simulink model "case_study_2"  (R2022a)
settings: Solver=VariableStepAuto  StartTime=0.0  StopTime=2000  RelTol=1e-3
settings Model: Creator=spinolam  LastModifiedBy=spinolam

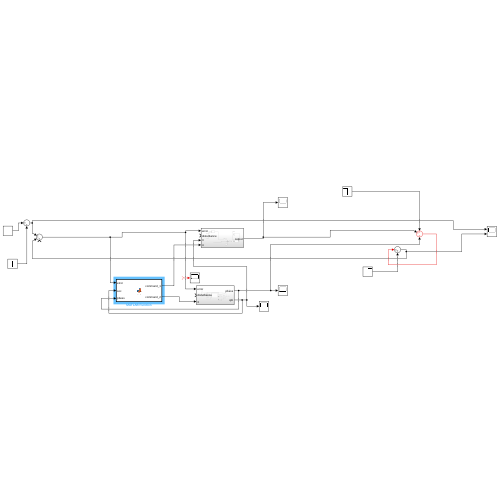
[thumbnail: Simulink's stored preview of the top-level diagram]
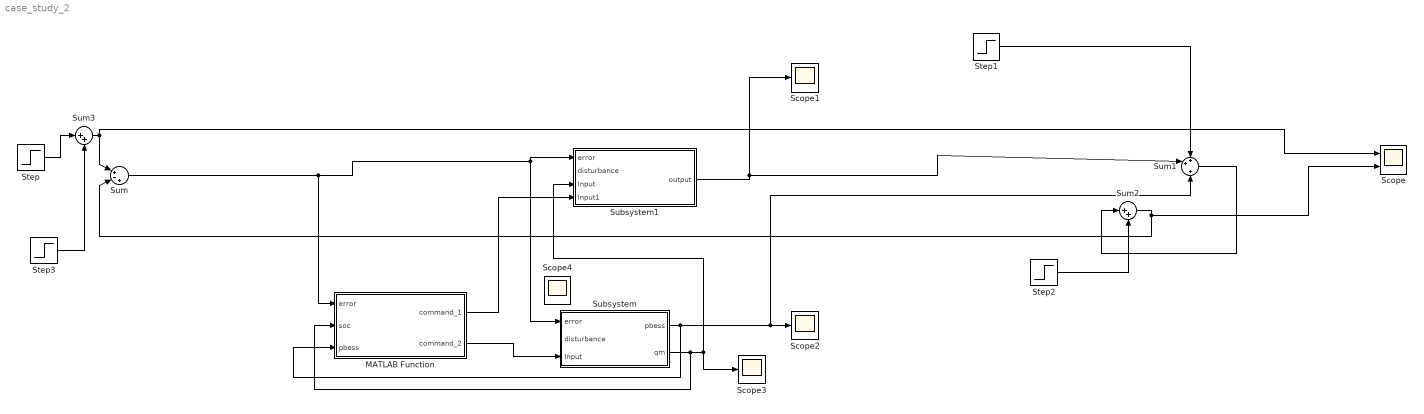
== system case_study_2 ==
  MATLAB Function : MATLAB Function  TreatAsAtomicUnit=on
  Scope : Scope  NumInputPorts=2
  Scope{1..4} (4 alike) : Scope
  Step : Step  Time=20  Before=1000  After=1300
  Step1 : Step  Time=100  After=-200
  Step2 : Step  Time=200  After=100
  Step3 : Step  Time=400  After=-100
  Subsystem : Subsystem
  Subsystem1 : Subsystem
  Sum : Sum  Inputs=|+-+
  Sum1 : Sum  Inputs=++|+
  Sum2 : Sum  Inputs=|++
  Sum3 : Sum  Inputs=|++
  wires:
  Step1/1 -> Sum1/1
  Sum1/1 -> Sum2/1
  Sum/1 -> MATLAB Function/1(error), Subsystem/1(error), Subsystem1/1(error)
  Subsystem1/1(output) -> Scope1/1, Sum1/2
  Subsystem/1(pbess) -> MATLAB Function/3(pbess), Sum1/3, Scope2/1
  Subsystem/2(qm) -> MATLAB Function/2(soc), Scope3/1, Subsystem1/3(Input)
  Sum2/1 -> Scope/2, Sum/2
  Step2/1 -> Sum2/2
  ? -> Scope4/1
  MATLAB Function/2(command_2) -> Subsystem/3(Input)
  MATLAB Function/1(command_1) -> Subsystem1/4(Input1)
  Step/1 -> Sum3/1
  Step3/1 -> Sum3/2
  Sum3/1 -> Sum/1, Scope/1

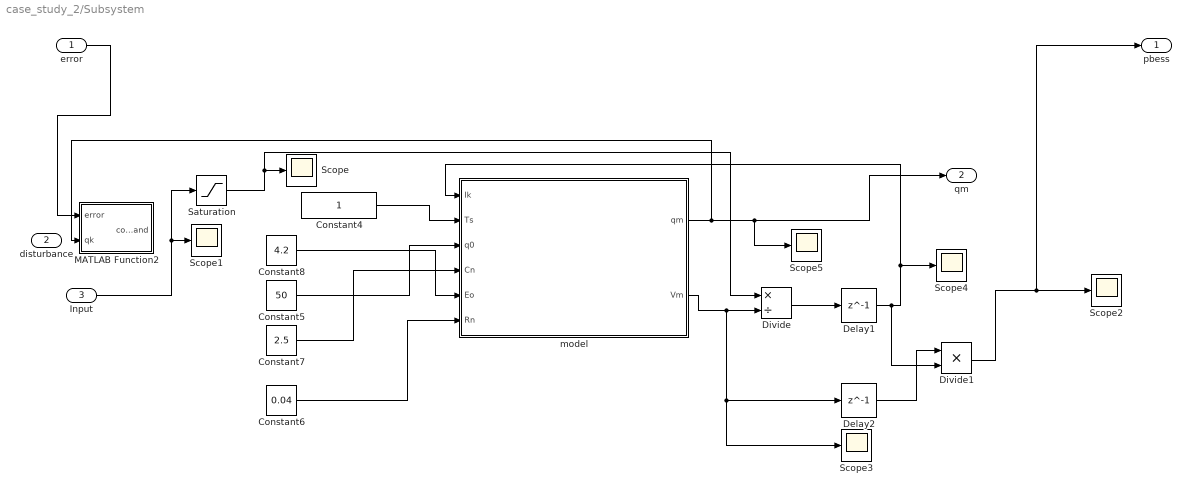
== system case_study_2/Subsystem ==
  error : Inport
  disturbance : Inport  Port=2
  Input : Inport  Port=3
  Constant4 : Constant  SampleTime=1
  Constant5 : Constant  Value=50
  Constant6 : Constant  Value=0.04
  Constant7 : Constant  Value=2.5
  Constant8 : Constant  Value=4.2
  Delay1 : Delay  DelayLength=1  InitialCondition=0  SampleTime=1
  Delay2 : Delay  DelayLength=1  InitialCondition=0  SampleTime=1
  Divide : Product  Inputs=*/
  Divide1 : Product  Inputs=**
  MATLAB Function2 : MATLAB Function  TreatAsAtomicUnit=on
  Saturation : Saturate  UpperLimit=140  LowerLimit=-140
  Scope{,1..5} (6 alike) : Scope
  model : MATLAB Function  TreatAsAtomicUnit=on  SystemSampleTime=1
  pbess : Outport
  qm : Outport  Port=2
  wires:
  Constant4/1 -> model/2(Ts)
  Constant6/1 -> model/6(Rn)
  Delay1/1 -> Divide1/2, Scope4/1, model/1(Ik)
  Divide1/1 -> pbess/1, Scope2/1
  Constant7/1 -> model/4(Cn)
  Divide/1 -> Delay1/1
  Delay2/1 -> Divide1/1
  Constant8/1 -> model/5(Eo)
  error/1 -> MATLAB Function2/1(error)
  model/2(Vm) -> Scope3/1, Delay2/1, Divide/2
  Constant5/1 -> model/3(q0)
  model/1(qm) -> MATLAB Function2/2(qk), Scope5/1, qm/1
  Saturation/1 -> Scope/1, Divide/1
  Input/1 -> Scope1/1, Saturation/1

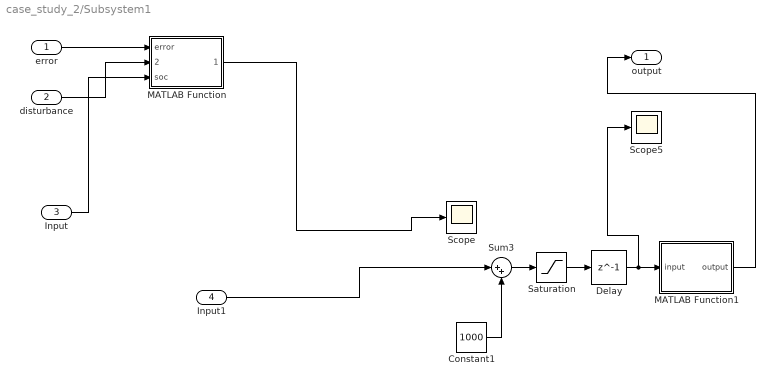
== system case_study_2/Subsystem1 ==
  error : Inport
  disturbance : Inport  Port=2
  Input : Inport  Port=3
  Input1 : Inport  Port=4
  Constant1 : Constant  Value=1000
  Delay : Delay  DelayLength=1  InitialCondition=1000  SampleTime=1
  MATLAB Function : MATLAB Function  TreatAsAtomicUnit=on
  MATLAB Function1 : MATLAB Function  TreatAsAtomicUnit=on
  Saturation : Saturate  UpperLimit=1500  LowerLimit=1000
  Scope : Scope
  Scope5 : Scope
  Sum3 : Sum  Inputs=|++
  output : Outport
  wires:
  MATLAB Function1/1(output) -> output/1
  MATLAB Function/1(command) -> Scope/1
  error/1 -> MATLAB Function/1(error)
  disturbance/1 -> MATLAB Function/2(disturbance)
  Sum3/1 -> Saturation/1
  Delay/1 -> Scope5/1, MATLAB Function1/1(input)
  Saturation/1 -> Delay/1
  Constant1/1 -> Sum3/2
  Input/1 -> MATLAB Function/3(soc)
  Input1/1 -> Sum3/1

== matlab function case_study_2/Subsystem1/MATLAB Function1 ==
  data: input input; output output
function output = fcn(input)
persistent output_old
alpha=0.5;
if isempty(output_old)
    output_old=1000;
end


output_new= (1-alpha)*output_old + alpha*input ;
output= output_old;
output_old=output_new;

== matlab function case_study_2/Subsystem1/MATLAB Function ==
  data: error input; command output; disturbance input; soc input
function command = fcn(error,disturbance,soc)
persistent z disturbance_old
kp=0.3; ki=0.3; kf=-0.5;
if isempty(z)
    z=0;
    disturbance_old=0;
end

if (error >0)
z=z+error;
else
    if soc <= 95
        z=z;
    else
        z=z+error;
    end
end
command= ki*z + kp*error +kf*disturbance_old -kf*disturbance;
disturbance_old = disturbance;

end

== matlab function case_study_2/MATLAB Function ==
  data: error input; command_1 output; soc input; command_2 output; pbess input
function [command_1,command_2] = fcn(error,soc, pbess)
persistent z1 z2 command_1_old command_2_old
kp_1=0.3; ki_1=0.3;
kp_2=0.1; ki_2=0.1;
if isempty(z1)
    z1=0;
    z2=0;
    command_1_old=0;
    command_2_old=0;
end
    command_1=command_1_old;
    z2=z2+error;
    command_2= ki_2*z2 + kp_2*error; 
    if error>0 || soc>= 95 || abs(pbess)>=140

    z1=z1+error;
    command_1= ki_1*z1 + kp_1*error ;
    
    end
    
    
    

    
    
    if (command_2 >0 && soc<= 5)
        command_2=0;
        z2=0;
    elseif(command_2 <0 && soc>= 95)
        command_2=0;
        z2=0;
    end
    command_1_old=command_1;
    command_2_old=command_2;

== matlab function case_study_2/Subsystem/MATLAB Function2 ==
  data: error input; command output; qk input
function command = fcn(error,qk)
persistent z disturbance_old
kp=0.1; ki=0.1; kf=-1;
if isempty(z)
    z=0;
    disturbance_old=0;
end

if error <0
 z=z+error;
else
    
end

command= ki*z + kp*error +0*kf*disturbance_old;
if (qk>=95 && command<=0)
    command=0;
    z=0;

elseif  (qk<=5 && command>=0)
    command=0;
    z=0;

end

== matlab function case_study_2/Subsystem/model ==
  data: Ik input; Ts input; qm output; Vm output; q0 input; Cn input; Eo input; Rn input
function [qm,Vm]= battery_twin(Ik,Ts, q0,Cn, Eo,Rn)

persistent qk Vk 
Ik=Ik;
% --- Parameters Battery ---
N=2;

% Parameters model Voc
K1=0.1;
K2=1;

% Parameters model Resistance
K3=0.25;
K4=0.04;
R0=0.005;

%Nominal capacity
Cr =N*Cn;


% --- initial states ----


if isempty(qk)
    qk=q0;
end
if isempty(Vk) 
    Vk=N*Eo; 
end


% --- dynamic model -----


q1 = qk - Ts*Ik*100*1/(3600*Cr);

Rint=N*(R0+K3/qk+K4/(100-qk))/2;
Eo=N*(Eo-K1*log(100-qk)-K2/qk);
Ek = Eo-(Rint)*Ik*1;
a=exp(-Ts/50);
V1 = a*Vk + (1-a)*Ek;

    %sensor model:
qm = qk; % + noise
Vm = Vk; % + noise

%updating z:

qk = q1;
Vk = V1;
